simulink model "HEV_powersplit_adapted"  (R2026a)
settings: Solver=VariableStepAuto  StopTime=DriveCycles(Drive_Cycle_Num).time(end)  FixedStep=Ts  AbsTol=1e-3  EnableMultiTasking=on
PreLoadFcn:
  | mdlDir = fileparts(get_param(bdroot,'FileName'));
  | if exist(mdlDir,'dir'), addpath(genpath(mdlDir)); end;
  | HEV_Model_HomeDir = mdlDir;
  | decimation = 1;
  | HEV_Model_PARAM;
  | HEV_SeriesParallel_param_detailed;
StartFcn:
  | tic;
StopFcn:
  | Elapsed_Sim_Time = toc;
undefined symbols (not defined in the file): AH, AH0, Drive_Cycle_Num, HEV_Param, Ld, Lq, p, psim, System, Ts, Vbat, VDC_VECT
libraries: fl_lib x70, nesl_utility x54, ee_lib x10, sdl_lib x6, eeTransforms x4, eePmsmCurrentController x2, eeGeneralControl x2, eePmsmCurrentReferenceGen x2, eePwmGeneratorTwoLevel x2, batteryecm_lib x1, Capacitors_lib x1, eePmsmTorqueEstimator x1
(part 2 of 3)

== system HEV_powersplit_adapted/Power Split Device/Sensor Carrier Shaft ==
  Ideal Rotational Motion Sensor : fl_lib/Mechanical/Mechanical Sensors/Ideal Rotational Motion Sensor  reference=foundation.enum.MeasurementReference.difference  acceleration_port=false  velocity_port=true  position_port=true  wrap_angle=simscape.enum.onoff.off  offset=0 rad
  Ideal Torque Sensor : fl_lib/Mechanical/Mechanical Sensors/Ideal Torque Sensor
  Mechanical Rotational Reference : fl_lib/Mechanical/Rotational Elements/Mechanical Rotational Reference
  PS-Simulink Converter : nesl_utility/PS-Simulink Converter  PhysicalDomain=network_engine_domain  SubClassName=ps_output  LeftPortType=input  RightPortType=output  PseudoPeriodic=off  Frequencies=[]  VectorFormat=1-D array  Unit=N*m  AffineConversion=off
  PS-Simulink Converter1 : nesl_utility/PS-Simulink Converter  PhysicalDomain=network_engine_domain  SubClassName=ps_output  LeftPortType=input  RightPortType=output  PseudoPeriodic=off  Frequencies=[]  VectorFormat=1-D array  Unit=rad/s  AffineConversion=off
  PG : PMIOPort  Side=Right
  Sh : PMIOPort  Port=2  Side=Left
  tag scope: Carrier_Spd_radps=global, Carrier_Trq_Nm=global
  wires:
  PS-Simulink Converter/1 -> [Carrier_Trq_Nm]  "Carrier torque (Nm)"
  PS-Simulink Converter1/1 -> [Carrier_Spd_radps]
  connections:
  Ideal Torque Sensor/RConn1 -- Sh/RConn1 -- Ideal Rotational Motion Sensor/RConn1
  Mechanical Rotational Reference/LConn1 -- Ideal Rotational Motion Sensor/LConn1
  PS-Simulink Converter/LConn1 -- Ideal Torque Sensor/RConn2
  PS-Simulink Converter1/LConn1 -- Ideal Rotational Motion Sensor/RConn2
  PG/RConn1 -- Ideal Torque Sensor/LConn1

== system HEV_powersplit_adapted/Power Split Device/Sensor Ring Shaft ==
  Ideal Rotational Motion Sensor : fl_lib/Mechanical/Mechanical Sensors/Ideal Rotational Motion Sensor  reference=foundation.enum.MeasurementReference.difference  acceleration_port=false  velocity_port=true  position_port=true  wrap_angle=simscape.enum.onoff.off  offset=0 rad
  Ideal Torque Sensor : fl_lib/Mechanical/Mechanical Sensors/Ideal Torque Sensor
  Mechanical Rotational Reference : fl_lib/Mechanical/Rotational Elements/Mechanical Rotational Reference
  PS-Simulink Converter : nesl_utility/PS-Simulink Converter  PhysicalDomain=network_engine_domain  SubClassName=ps_output  LeftPortType=input  RightPortType=output  PseudoPeriodic=off  Frequencies=[]  VectorFormat=1-D array  Unit=N*m  AffineConversion=off
  PS-Simulink Converter1 : nesl_utility/PS-Simulink Converter  PhysicalDomain=network_engine_domain  SubClassName=ps_output  LeftPortType=input  RightPortType=output  PseudoPeriodic=off  Frequencies=[]  VectorFormat=1-D array  Unit=rad/s  AffineConversion=off
  PG : PMIOPort  Side=Right
  Sh : PMIOPort  Port=2  Side=Left
  tag scope: Ring_Spd_radps=global, Ring_Trq_Nm=global
  wires:
  PS-Simulink Converter/1 -> [Ring_Trq_Nm]  "Ring  torque (Nm)"
  PS-Simulink Converter1/1 -> [Ring_Spd_radps]  "Ring speed (rad/s)"
  connections:
  Ideal Rotational Motion Sensor/RConn1 -- PG/RConn1 -- Ideal Torque Sensor/RConn1
  Sh/RConn1 -- Ideal Torque Sensor/LConn1
  PS-Simulink Converter/LConn1 -- Ideal Torque Sensor/RConn2
  Mechanical Rotational Reference/LConn1 -- Ideal Rotational Motion Sensor/LConn1
  PS-Simulink Converter1/LConn1 -- Ideal Rotational Motion Sensor/RConn2

== system HEV_powersplit_adapted/Power Split Device/Sensor Sun Shaft ==
  Ideal Rotational Motion Sensor : fl_lib/Mechanical/Mechanical Sensors/Ideal Rotational Motion Sensor  reference=foundation.enum.MeasurementReference.difference  acceleration_port=false  velocity_port=true  position_port=true  wrap_angle=simscape.enum.onoff.off  offset=0 rad
  Ideal Torque Sensor : fl_lib/Mechanical/Mechanical Sensors/Ideal Torque Sensor
  Mechanical Rotational Reference : fl_lib/Mechanical/Rotational Elements/Mechanical Rotational Reference
  PS-Simulink Converter : nesl_utility/PS-Simulink Converter  PhysicalDomain=network_engine_domain  SubClassName=ps_output  LeftPortType=input  RightPortType=output  PseudoPeriodic=off  Frequencies=[]  VectorFormat=1-D array  Unit=N*m  AffineConversion=off
  PS-Simulink Converter1 : nesl_utility/PS-Simulink Converter  PhysicalDomain=network_engine_domain  SubClassName=ps_output  LeftPortType=input  RightPortType=output  PseudoPeriodic=off  Frequencies=[]  VectorFormat=1-D array  Unit=rad/s  AffineConversion=off
  PG : PMIOPort  Side=Right
  Sh : PMIOPort  Port=2  Side=Left
  tag scope: Sun_Spd_radps=global, Sun_Trq_Nm=global
  wires:
  PS-Simulink Converter1/1 -> [Sun_Spd_radps]
  PS-Simulink Converter/1 -> [Sun_Trq_Nm]  "Sun_Trq_Nm"
  connections:
  Sh/RConn1 -- Ideal Torque Sensor/LConn1
  PS-Simulink Converter1/LConn1 -- Ideal Rotational Motion Sensor/RConn2
  PS-Simulink Converter/LConn1 -- Ideal Torque Sensor/RConn2
  Mechanical Rotational Reference/LConn1 -- Ideal Rotational Motion Sensor/LConn1
  PG/RConn1 -- Ideal Torque Sensor/RConn1 -- Ideal Rotational Motion Sensor/RConn1

== system HEV_powersplit_adapted/Scopes/Drivetrain Scopes ==
  Speed (rad/s) : Scope  NumInputPorts=3
      settings: ActiveDisplayYMinimum=-100  ActiveDisplayYMaximum=500  DataLoggingMaxPoints=100  DataLoggingDecimation=decimation  DataLoggingVariableName=ScopeData2
  Torque (Nm) : Scope  Commented=on  NumInputPorts=3
      settings: ActiveDisplayYMinimum=-50  ActiveDisplayYMaximum=150  DataLoggingMaxPoints=100  DataLoggingDecimation=decimation  DataLoggingVariableName=ScopeData4
  wires:
  [Ring_Spd_radps] -> Speed (rad/s)/2  "Ring speed (rad/s) - motor"
  [Sun_Spd_radps] -> Speed (rad/s)/3  "Sun speed (rad/s) - generator"
  [Ring_Trq_Nm] -> Torque (Nm)/2  "Ring torque (Nm) - motor"
  [Carrier_Spd_radps] -> Speed (rad/s)/1  "Carrier speed (rad/s) - engine (ICE)"
  [Sun_Trq_Nm] -> Torque (Nm)/3  "Sun torque (Nm) - generator"
  [Carrier_Trq_Nm] -> Torque (Nm)/1  "Carrier torque (Nm) - engine (ICE)"

== system HEV_powersplit_adapted/Scopes/Power Calculation2 ==
  Spd : Inport
  Tq : Inport  Port=2
  Gain4 : Gain  Gain=1/1000
  Product2 : Product
  rpm2rad/s : Gain  Gain=pi/30
  Power : Outport  VectorParamsAs1DForOutWhenUnconnected=off
  wires:
  Spd/1 -> rpm2rad/s/1
  Gain4/1 -> Power/1
  Product2/1 -> Gain4/1
  Tq/1 -> Product2/2
  rpm2rad/s/1 -> Product2/1

== system HEV_powersplit_adapted/Scopes/Power Calculation ==
  Spd : Inport
  Tq : Inport  Port=2
  Gain4 : Gain  Gain=1/1000
  Product2 : Product
  rpm2rad/s : Gain  Gain=pi/30
  Power : Outport  VectorParamsAs1DForOutWhenUnconnected=off
  wires:
  Spd/1 -> rpm2rad/s/1
  Gain4/1 -> Power/1
  Product2/1 -> Gain4/1
  Tq/1 -> Product2/2
  rpm2rad/s/1 -> Product2/1

== system HEV_powersplit_adapted/Vehicle/Sensor Speed and Power ==
  Ideal Rotational Motion Sensor : fl_lib/Mechanical/Mechanical Sensors/Ideal Rotational Motion Sensor  reference=foundation.enum.MeasurementReference.difference  acceleration_port=false  velocity_port=true  position_port=true  wrap_angle=simscape.enum.onoff.off  offset=0 rad
  Ideal Torque Sensor : fl_lib/Mechanical/Mechanical Sensors/Ideal Torque Sensor
  Mechanical Rotational Reference : fl_lib/Mechanical/Rotational Elements/Mechanical Rotational Reference
  PS-Simulink Converter : nesl_utility/PS-Simulink Converter  PhysicalDomain=network_engine_domain  SubClassName=ps_output  LeftPortType=input  RightPortType=output  PseudoPeriodic=off  Frequencies=[]  VectorFormat=1-D array  Unit=N*m  AffineConversion=off
  PS-Simulink Converter1 : nesl_utility/PS-Simulink Converter  PhysicalDomain=network_engine_domain  SubClassName=ps_output  LeftPortType=input  RightPortType=output  PseudoPeriodic=off  Frequencies=[]  VectorFormat=1-D array  Unit=rad/s  AffineConversion=off
  Product : Product  RndMeth=Zero
  W2kW : Gain  Gain=0.001
  B : PMIOPort  Side=Left
  F : PMIOPort  Port=2  Side=Right
  tag scope: P_dem=global
  wires:
  W2kW/1 -> [P_dem]
  Product/1 -> W2kW/1
  PS-Simulink Converter/1 -> Product/1
  PS-Simulink Converter1/1 -> Product/2
  connections:
  Mechanical Rotational Reference/LConn1 -- Ideal Rotational Motion Sensor/RConn1
  Ideal Rotational Motion Sensor/LConn1 -- F/RConn1 -- Ideal Torque Sensor/RConn1
  B/RConn1 -- Ideal Torque Sensor/LConn1
  PS-Simulink Converter/LConn1 -- Ideal Torque Sensor/RConn2
  PS-Simulink Converter1/LConn1 -- Ideal Rotational Motion Sensor/RConn2

== system HEV_powersplit_adapted/Control/Engine Speed Controller/Engine Running ==
  note: Manual enable for control logic
  ICE_Enable : Inport
  Constant : Constant
  Select Logic : ManualSwitch  CurrentSetting=0
  Engine Running : Outport  VectorParamsAs1DForOutWhenUnconnected=off
  tag scope: engine_running=global
  wires:
  ICE_Enable/1 -> Select Logic/2
  Select Logic/1 -> Engine Running/1, [engine_running]
  Constant/1 -> Select Logic/1

== system HEV_powersplit_adapted/Control/Generator Controller/Enable Torque Demand ==
  Gen_Enable : Inport
  TrqDemCtrl : Inport  Port=2
  20Hz Lowpass Filter : TransferFcn  Denominator=[1/(2*pi*20) 1]
  Product : Product  RndMeth=Zero
  Select Logic : ManualSwitch  CurrentSetting=0
  G_Trq_Dem : Outport  VectorParamsAs1DForOutWhenUnconnected=off
  wires:
  Gen_Enable/1 -> 20Hz Lowpass Filter/1
  TrqDemCtrl/1 -> Product/2, Select Logic/2
  20Hz Lowpass Filter/1 -> Product/1
  Select Logic/1 -> G_Trq_Dem/1
  Product/1 -> Select Logic/1

== system HEV_powersplit_adapted/Control/Generator Controller/Speed controller ==
  note: This loop controls motor speed. The maximum value for V_wref is 5 volts,
      | which is equivalent to a speed demand of 10000rpm.
  Wref : Inport
  W : Inport  Port=2
  20Hz Lowpass Filter : TransferFcn  Denominator=[1/(2*pi*20) 1]
  Gen RPM to V : Gain  Gain=5/10000
  Ki : Gain  Gain=HEV_Param.Control.Gen.Ki
  Kp : Gain  Gain=HEV_Param.Control.Gen.Kp
  Limits [-5,5] : Integrator  ExternalReset=either  LimitOutput=on  UpperSaturationLimit=5  LowerSaturationLimit=-5
  Sum : Sum  Inputs=-+|
  Sum1 : Sum  Inputs=++|
  Volts/Nm : Gain  Gain=400/5
  "[-5,5]" : Saturate  UpperLimit=5  LowerLimit=-5
  rpm2volts : Gain  Gain=5/10000
  Tref : Outport  VectorParamsAs1DForOutWhenUnconnected=off
  wires:
  Sum/1 -> Ki/1, Kp/1
  [engine_running] -> Limits [-5,5]/2
  20Hz Lowpass Filter/1 -> Sum/1
  Limits [-5,5]/1 -> Sum1/1
  Kp/1 -> Sum1/2
  Ki/1 -> Limits [-5,5]/1
  Sum1/1 -> "[-5,5]"/1
  W/1 -> Gen RPM to V/1
  Wref/1 -> rpm2volts/1
  "[-5,5]"/1 -> Volts/Nm/1
  rpm2volts/1 -> Sum/2
  Gen RPM to V/1 -> 20Hz Lowpass Filter/1
  Volts/Nm/1 -> Tref/1

== system HEV_powersplit_adapted/Control/Generator Controller/Subsystem1 ==
  In1 : Inport
  Gen_RPM_Dem : Outport  VectorParamsAs1DForOutWhenUnconnected=off
  wires:
  In1/1 -> Gen_RPM_Dem/1

== system HEV_powersplit_adapted/Control/Motor Controller/Enable Torque Demand ==
  Mot_Enable : Inport
  TrqDemCtrl : Inport  Port=2
  20Hz Lowpass Filter : TransferFcn  Commented=on  Denominator=[1/(2*pi*10) 1]
  Product : Product  RndMeth=Zero
  Select Logic : ManualSwitch  CurrentSetting=0
  TrqDem : Outport  VectorParamsAs1DForOutWhenUnconnected=off
  wires:
  Mot_Enable/1 -> 20Hz Lowpass Filter/1
  TrqDemCtrl/1 -> Product/2, Select Logic/2
  Product/1 -> Select Logic/1
  20Hz Lowpass Filter/1 -> Product/1
  Select Logic/1 -> TrqDem/1

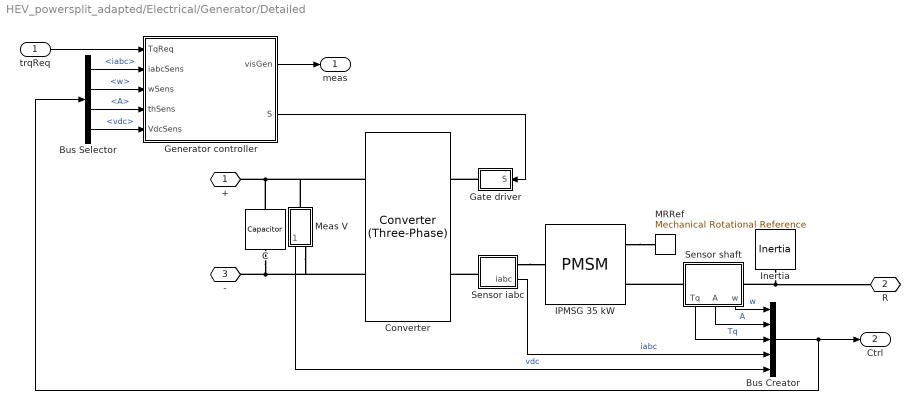
== system HEV_powersplit_adapted/Electrical/Generator/Detailed ==
  trqReq : Inport
  Bus Creator : BusCreator  Inputs=5
  Bus Selector : BusSelector  OutputSignals=iabc,w,A,vdc
  C : fl_lib/Electrical/Electrical Elements/Capacitor  c=Cdc F  r=1e-6 Ohm  g=0 1/Ohm  i_specify=off  i_priority=None  i=0 A  i_nominal_specify=off  i_nominal_value=1  i_nominal_unit=A  v_specify=off  v_priority=None  v=0 V  v_nominal_specify=off  v_nominal_value=1  v_nominal_unit=V  vc_specify=on  vc_priority=None  vc=Vbat*1.4 V  vc_nominal_specify=off  vc_nominal_value=1  vc_nominal_unit=V
  Converter : ee_lib/Semiconductors & Converters/Converters/Converter (Three-Phase)  port_option=ee.enum.threePhasePort.composite  fidelity_option=ee.enum.converters.fidelity.detailed  device_type=2  showThermalPort=false  K=0  Vth=0.5 V  Vgt=1 V  Vgt_off=-1 V  Ih=1 A  Vf=0.8 V  Ron=0.001 Ohm  Rds=0.001 Ohm  Goff=1e-5 1/Ohm  Eon_scalar=22.86e-3 J  Eoff_scalar=17.14e-3 J  Eoff_natural_commutation=10e-3 J  Voff=300 V  Iout_scalar=600 A  onCurrentMeasDelay=0 s  useCurrentFromPreviousCycle=false  useVoltageFromPreviousCycle=false  diode_param=2  diode_Vf=0.8 V  diode_Ron=0.001 Ohm  diode_Goff=1e-5 1/Ohm  diode_C=50 nF  diode_iRM=-235 A  diode_iF=300 A  diode_idot=-50 A/us  diode_trr_param=1  diode_trr_factor=3  diode_trr=15 us  diode_Qrr=1.5e+3 s*uA  diode_rec_loss_model=ee.enum.diode.reverseRecoveryModel.fixed  diode_ErecVal=0 J  diode_scaleWithIandV=false  diode_ErecMat=zeros(2, 3) J  diode_TjrecVec=[298.15, 398.15] K  diode_IfrecVec=[.1, 1, 10] A  diode_IrecVal=10 A  diode_VrecVal=10 V  diode_tFilter=1 / 1000 / 100 s  thermal_network_parameterization=ee.enum.thermalNetworkTopology.external  Rth=[.08, .5] K/W  Rth_Cauer=[.08, .1, .5] K/W  Rth_Foster=[.08, .14, .22, .16] K/W  thermal_mass_parameterization=ee.enum.thermalNetwork.timeconstant  thermal_mass=[.01, .5] J/K  thermal_mass_Cauer=[.01, .1, .5] J/K  thermal_mass_Foster=[.001, .005, .05, .5] J/K  thermal_time_constant=[.001, .2] s  thermal_time_constant_Cauer=[.001, .1, .2] s  thermal_time_constant_Foster=[7e-05, .0007, .01, .08] s  thermal_mass_initial_temperatures=[25, 25] degC  thermal_mass_initial_temperatures_Cauer=[25, 25, 25] degC  junction_thermal_mass=0.01 J/K  Tvec_initial_Foster=[25, 25, 25, 25] degC  snubber_type=0  Cs=1e-7 F  Rs=0.1 Ohm  Vce_loss=[0, 150, 300] V
      settings: LogSimulationData=on
  Gate driver : Subsystem
  Generator controller : Subsystem
  IPMSG 35 kW : ee_lib/Electromechanical/Permanent Magnet/PMSM  port_option=ee.enum.threePhasePort.composite  winding_type=ee.enum.statorconnection.wye  machine_param=ee.enum.pmsm.parameterization.constant  nPolePairs=p  pmflux_param=1  pm_flux_linkage=psim Wb  torque_constant=0.18 N*m/A  back_emf_constant=0.18 V/(rad/s)  stator_param=1  Ld=Ld H  Lq=Lq H  idVec=[-200, 0, 200] A  iqVec=[-200, 0, 200] A  LdMatrix=0.0002 * ones(3, 3) H  LqMatrix=0.0002 * ones(3, 3) H  PmMatrix=0.1 * ones(3, 3) Wb  ktMatrix=0.18 * ones(3, 3) N*m/A  keMatrix=0.18 * ones(3, 3) V/(rad/s)  L0=L0 H  Ls=0.0002 H  Lm=0.00002 H  Ms=0.00002 H  Rs=Rs Ohm  zero_sequence=ee.enum.park.zerosequence.exclude  axes_param=1  loss_param=ee.enum.ironloss.none  losses_oc=[0, 0, 0] W  losses_sc=[0, 0, 0] W  f_losses=60 Hz  Isc_losses=95 A  J=0.01 kg*m^2  lam=0 N*m/(rad/s)  i_d_specify=off  i_d_priority=None  i_d=0 A  i_d_nominal_specify=off  i_d_nominal_value=1  i_d_nominal_unit=A  i_q_specify=off  i_q_priority=None  i_q=0 A  i_q_nominal_specify=off  i_q_nominal_value=1  i_q_nominal_unit=A  torque_specify=off  torque_priority=None  torque=0 N*m  torque_nominal_specify=off  torque_nominal_value=1  torque_nominal_unit=N*m  angular_velocity_specify=on  angular_velocity_priority=Low  angular_velocity=0 rpm  angular_velocity_nominal_specify=off  angular_velocity_nominal_value=1  angular_velocity_nominal_unit=rpm  angular_position_specify=off  angular_position_priority=None  angular_position=0 deg  angular_position_nominal_specify=off  angular_position_nominal_value=1  angular_position_nominal_unit=deg  alpha=3.93e-3 1/K  alpha_flux=-0.001 1/K  Tmeas=298.15 K  stator_thermal_mass=100 J/K  rotor_thermal_mass=200 J/K  Rm_percent_rotor=90  Rd_percent_rotor=30  temperatureA_specify=off  temperatureA_priority=High  temperatureA=25 degC  temperatureA_nominal_specify=off  temperatureA_nominal_value=1  temperatureA_nominal_unit=degC  temperatureB_specify=off  temperatureB_priority=High  temperatureB=25 degC  temperatureB_nominal_specify=off  temperatureB_nominal_value=1  temperatureB_nominal_unit=degC  temperatureC_specify=off  temperatureC_priority=High  temperatureC=25 degC  temperatureC_nominal_specify=off  temperatureC_nominal_value=1  temperatureC_nominal_unit=degC  temperatureR_specify=off  temperatureR_priority=High  temperatureR=25 degC  temperatureR_nominal_specify=off  temperatureR_nominal_value=1  temperatureR_nominal_unit=degC
      settings: LogSimulationData=on  InternalSimscapePortConfiguration="{\"Bottom\":[],\"Left\":[{\"id\":\"N\",\"label\":\"~\",\"type\":\"foundation.electrical.three_phase\"}],\"Right\":[{\"id\":\"R\",\"label\":\"R\",\"type\":\"foundation.mechanical.rotational.rotational\"},{\"id\":\"C\",\"label\":\"C\",\"type\":\"foundation.mechanical.rotational.rotational\"}],\"Top\":[]}"
  Inertia : fl_lib/Mechanical/Rotational Elements/Inertia  inertia=0.1 kg*m^2  num_ports=foundation.enum.numPorts2.one  w_specify=on  w_priority=Low  w=0 rad/s  w_nominal_specify=off  w_nominal_value=1  w_nominal_unit=rad/s  t_specify=off  t_priority=None  t=0 N*m  t_nominal_specify=off  t_nominal_value=1  t_nominal_unit=N*m
  MRRef : fl_lib/Mechanical/Rotational Elements/Mechanical Rotational Reference
  Meas V : Subsystem
  Sensor iabc : Subsystem
      settings: PortSchema="{\"entries\":[{\"content\":{\"sides\":[{\"content\":{\"connectorIds\":[\"LConn1\"]},\"type\":\"ConnectorPlacement.EquallySpacedRectSide\",\"uuid\":\"bc3757cc-4537-444e-89af-7b7d8c8c1fa7\"},{\"content\":{\"connectorIds\":[\"RConn1\",\"Out1\"],\"side\":\"RIGHT\"},\"type\":\"ConnectorPlacement.EquallySpacedRectSide\",\"uuid\":\"908bf4c4-26f6-4d8a-bcf8-68236027f5f8\"},{\"content\":{\"connectorIds\":[],\"side\":\"TOP\"},\"type\":\"ConnectorPlacement.EquallySpacedRectSide\",\"uuid\":\"33f228db-ba47-4718-96dc-a72de309ae8c\"}]},\"type\":\"ConnectorPlacement.EquallySpacedConnector\",\"uuid\":\"345f3578-0572-4e64-b2f3-84728129a12d\"}],\"packageUris\":[\"http://schema.mathworks.com/mf0/Connector/R2020b\"],\"version\":\"1.0\"}"
  Sensor shaft : Subsystem
      settings: PortSchema="{\"entries\":[{\"content\":{\"sides\":[{\"content\":{\"connectorIds\":[\"LConn1\"]},\"type\":\"ConnectorPlacement.EquallySpacedRectSide\",\"uuid\":\"0db9bac0-0ae1-4d98-a677-466f391c258c\"},{\"content\":{\"connectorIds\":[\"RConn1\"],\"side\":\"RIGHT\"},\"type\":\"ConnectorPlacement.EquallySpacedRectSide\",\"uuid\":\"8934243c-3b81-4e7c-b06c-d9d72f311b85\"},{\"content\":{\"connectorIds\":[],\"side\":\"TOP\"},\"type\":\"ConnectorPlacement.EquallySpacedRectSide\",\"uuid\":\"85d02103-2e2c-4b6a-97e8-ffc8c956f28d\"},{\"content\":{\"connectorIds\":[\"Out1\",\"Out2\",\"Out3\"],\"side\":\"BOTTOM\"},\"type\":\"ConnectorPlacement.EquallySpacedRectSide\",\"uuid\":\"2e7d2385-134f-4bd8-b3f4-60582ce11538\"}]},\"type\":\"ConnectorPlacement.EquallySpacedConnector\",\"uuid\":\"45a37dc1-16bf-4b9c-909e-727af625c5bc\"}],\"packageUris\":[\"http://schema.mathworks.com/mf0/Connector/R2020b\"],\"version\":\"1.0\"}"
  + : PMIOPort  Side=Left
  R : PMIOPort  Port=2  Side=Right
  - : PMIOPort  Port=3  Side=Left
  meas : Outport
  Ctrl : Outport  Port=2
  wires:
  Generator controller/1(visGen) -> meas/1
  trqReq/1 -> Generator controller/1(TqReq)
  Bus Selector/2 -> Generator controller/3(wSens)  "<w>"
  Bus Selector/4 -> Generator controller/5(VdcSens)  "<vdc>"
  Bus Selector/3 -> Generator controller/4(thSens)  "<A>"
  Bus Selector/1 -> Generator controller/2(iabcSens)  "<iabc>"
  Bus Creator/1 -> Bus Selector/1, Ctrl/1
  Sensor shaft/1(Tq) -> Bus Creator/3  "Tq"
  Sensor iabc/1(iabc) -> Bus Creator/4  "iabc"
  Meas V/1(Vdc) -> Bus Creator/5  "vdc"
  Sensor shaft/3(w) -> Bus Creator/1  "w"
  Sensor shaft/2(A) -> Bus Creator/2  "A"
  Generator controller/2(S) -> Gate driver/1(S)
  connections:
  C/LConn1 -- Meas V/LConn1 -- Converter/RConn1 -- +/RConn1
  Sensor iabc/RConn1 -- IPMSG 35 kW/LConn1
  Sensor iabc/LConn1 -- Converter/LConn2
  Inertia/LConn1 -- R/RConn1 -- Sensor shaft/RConn1
  Sensor shaft/LConn1 -- IPMSG 35 kW/RConn1
  Gate driver/RConn1 -- Converter/LConn1
  C/RConn1 -- -/RConn1 -- Converter/RConn2 -- Meas V/RConn1
  IPMSG 35 kW/RConn2 -- MRRef/LConn1

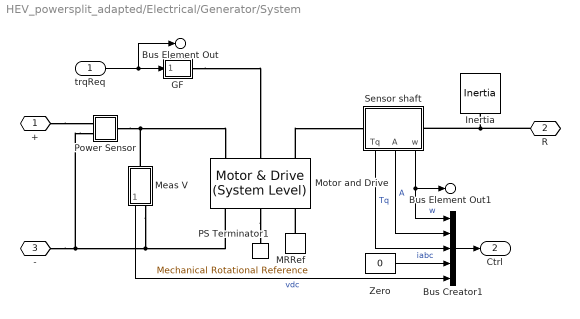
== system HEV_powersplit_adapted/Electrical/Generator/System ==
  trqReq : Inport
  Bus Creator1 : BusCreator  Inputs=5
  GF : Subsystem
      mask Display: disp('GF')
  Inertia : fl_lib/Mechanical/Rotational Elements/Inertia  inertia=HEV_Param.Generator.Shaft_Inertia kg*m^2  num_ports=foundation.enum.numPorts2.one  w_specify=on  w_priority=None  w=0 rad/s  w_nominal_specify=off  w_nominal_value=1  w_nominal_unit=rad/s  t_specify=off  t_priority=High  t=0 N*m  t_nominal_specify=off  t_nominal_value=1  t_nominal_unit=N*m
  MRRef : fl_lib/Mechanical/Rotational Elements/Mechanical Rotational Reference
  Meas V : Subsystem
  Motor and Drive : ee_lib/Electromechanical/Motor & Drive (System Level)  torque_speed_param=1  overtorque_param=ee.enum.electromech.overtorque.no  T_t=HEV_Param.Generator.TorqSpdLUT.TorqueNm N*m  T_t_intermittent=[.36, .32, .28, 0] N*m  T_t_2D=[.09, .09, .09; .08, .08, .08; .07, .07, .07; 0, 0, 0] N*m  T_t_intermittent_2D=[.36, .36, .36; .32, .32, .32; .28, .28, .28; 0, 0, 0] N*m  w_t=HEV_Param.Generator.TorqSpdLUT.SpeedRPM rpm  vdc_t=[6, 12, 24] V  torque_max=0.1 N*m  power_max=30 W  torque_max_intermittent=0.4 N*m  power_max_intermittent=120 W  time_overtorque=30 s  time_recover=60 s  Tc=HEV_Param.Generator.TorqueControl_TimeConst/2 s  EnableSwitch=simscape.enum.onoff.off  losses_param=1  eff=90  w_eff=2000 rpm  T_eff=200 N*m  Piron=0 W  Pbase=HEV_Param.Generator.TorqIndep_Elec_Loss W  w_eff_vec=[-8000 -4000 0 4000 8000] rpm  T_eff_vec=[0 0.03 0.06 0.09] N*m  v_eff_vec=[100, 250, 400] V  losses_mat=[1.49 1.67 2.21 3.10; 0.42 0.69 1.14 2.03; 0.06 0.24 0.78 1.68; 0.42 0.69 1.14 2.03; 1.49 1.67 2.21 3.10] W  efficiency_mat=[95 95 95 95; 95 95 95 95; 95 95 95 95; 95 95 95 95; 95 95 95 95]  losses_mat_3D=ones(5, 4, 3) W  efficiency_mat_3D=95 * ones(5, 4, 3)  Res=HEV_Param.Generator.Series_Resistance Ohm  J=0 kg*m^2  lam=HEV_Param.Generator.Damping N*m/(rad/s)  speed0=0 rpm  faulted_specify=off  faulted_priority=None  faulted=0  faulted_nominal_specify=off  faulted_nominal_value=1  faulted_nominal_unit=1  isSwitchedOff_specify=off  isSwitchedOff_priority=None  isSwitchedOff=0  isSwitchedOff_nominal_specify=off  isSwitchedOff_nominal_value=1  isSwitchedOff_nominal_unit=1  torqueLimitContinuous_specify=off  torqueLimitContinuous_priority=None  torqueLimitContinuous=0 N*m  torqueLimitContinuous_nominal_specify=off  torqueLimitContinuous_nominal_value=1  torqueLimitContinuous_nominal_unit=N*m  TabulateLossesForMultipleTemperatures=false  alpha=3.93e-3 1/K  Tmeas=25 degC  TmeasVec=[25, 75, 125] degC  Tmeas2=125 degC  losses_mat_T2=[1.49, 1.74, 2.49, 3.74; .42, .67, 1.42, 2.67; .06, .31, 1.06, 2.31; .42, .67, 1.42, 2.67; 1.49, 1.74, 2.49, 3.74] W  efficiency_mat_T2=[95, 95, 95, 95; 95, 95, 95, 95; 95, 95, 95, 95; 95, 95, 95, 95; 95, 95, 95, 95]  losses_mat_3D_T2=ones(5, 4, 3) W  efficiency_mat_3D_T2=95 * ones(5, 4, 3)  lossesMatMultipleTemperatures=ones(5, 4, 3) W  efficiencyMatMultipleTemperatures=95 * ones(5, 4, 3)  lossesMat4DMultipleTemperatures=ones(5, 4, 3, 3) W  efficiencyMat4DMultipleTemperatures=95 * ones(5, 4, 3, 3)  thermal_mass=100 J/K  initial_temperature=25 degC
  PS Terminator1 : fl_lib/Physical Signals/Sinks/PS Terminator
  Power Sensor : Subsystem
      mask Display: disp('S')
  Sensor shaft : Subsystem
      settings: PortSchema="{\"entries\":[{\"content\":{\"sides\":[{\"content\":{\"connectorIds\":[\"LConn1\"]},\"type\":\"ConnectorPlacement.EquallySpacedRectSide\",\"uuid\":\"0db9bac0-0ae1-4d98-a677-466f391c258c\"},{\"content\":{\"connectorIds\":[\"RConn1\"],\"side\":\"RIGHT\"},\"type\":\"ConnectorPlacement.EquallySpacedRectSide\",\"uuid\":\"8934243c-3b81-4e7c-b06c-d9d72f311b85\"},{\"content\":{\"side\":\"TOP\"},\"type\":\"ConnectorPlacement.EquallySpacedRectSide\",\"uuid\":\"85d02103-2e2c-4b6a-97e8-ffc8c956f28d\"},{\"content\":{\"connectorIds\":[\"Out1\",\"Out2\",\"Out3\"],\"side\":\"BOTTOM\"},\"type\":\"ConnectorPlacement.EquallySpacedRectSide\",\"uuid\":\"2e7d2385-134f-4bd8-b3f4-60582ce11538\"}]},\"type\":\"ConnectorPlacement.EquallySpacedConnector\",\"uuid\":\"45a37dc1-16bf-4b9c-909e-727af625c5bc\"}],\"packageUris\":[\"http://schema.mathworks.com/mf0/Connector/R2020b\"],\"version\":\"1.0\"}"
  Zero : Constant  Value=0  OutDataTypeStr=Inherit: Inherit via back propagation
  + : PMIOPort  Side=Left
  R : PMIOPort  Port=2  Side=Right
  - : PMIOPort  Port=3  Side=Left
  Bus Element Out : Outport  PortName=meas  Element=TqRef
  Bus Element Out1 : Outport  PortName=meas  Element=Spd
  Ctrl : Outport  Port=2  VectorParamsAs1DForOutWhenUnconnected=off
  wires:
  Meas V/1(Vdc) -> Bus Creator1/5  "vdc"
  Bus Creator1/1 -> Ctrl/1
  Sensor shaft/3(w) -> Bus Element Out1/1, Bus Creator1/1  "w"
  Zero/1 -> Bus Creator1/4  "iabc"
  Sensor shaft/1(Tq) -> Bus Creator1/3  "Tq"
  Sensor shaft/2(A) -> Bus Creator1/2  "A"
  trqReq/1 -> Bus Element Out/1, GF/1(In1)
  connections:
  R/RConn1 -- Sensor shaft/RConn1 -- Inertia/LConn1
  Power Sensor/LConn2 -- -/RConn1 -- Motor and Drive/RConn1 -- Meas V/RConn1
  +/RConn1 -- Power Sensor/LConn1
  Power Sensor/RConn1 -- Motor and Drive/LConn1 -- Meas V/LConn1
  GF/RConn1 -- Motor and Drive/LConn2
  Motor and Drive/RConn2 -- PS Terminator1/LConn1
  MRRef/LConn1 -- Motor and Drive/RConn3
  Motor and Drive/LConn3 -- Sensor shaft/LConn1

== system HEV_powersplit_adapted/Electrical/Generic/Measurements1 ==
  Bus Creator : BusCreator  Inputs=4
  Calc Pct : Gain  Gain=1/AH*100
  Calculate battery power & charge : Subsystem
  Gain : Gain  Gain=1/100
  PS-Simulink Converter1 : nesl_utility/PS-Simulink Converter  PhysicalDomain=network_engine_domain  SubClassName=ps_output  LeftPortType=input  RightPortType=output  PseudoPeriodic=off  Frequencies=[]  VectorFormat=1-D array  Unit=V  AffineConversion=off
  PS-Simulink Converter2 : nesl_utility/PS-Simulink Converter  PhysicalDomain=network_engine_domain  SubClassName=ps_output  LeftPortType=input  RightPortType=output  PseudoPeriodic=off  Frequencies=[]  VectorFormat=1-D array  Unit=A  AffineConversion=off
  VBatt : PMIOPort  Side=Left
  IBatt : PMIOPort  Port=2  Side=Left
  Batt_Ah : Outport  VectorParamsAs1DForOutWhenUnconnected=off
  Batt_Meas : Outport  Port=2  VectorParamsAs1DForOutWhenUnconnected=off
  SOC : Outport  Port=3
  wires:
  Bus Creator/1 -> Batt_Meas/1
  PS-Simulink Converter2/1 -> Bus Creator/4  "Current (A)"
  PS-Simulink Converter1/1 -> Bus Creator/3  "Voltage (V)"
  Calc Pct/1 -> Gain/1, Bus Creator/2  "SOC (%)"
  Calculate battery power & charge/1(Ah) -> Batt_Ah/1, Calc Pct/1, Bus Creator/1  "Batt_Ah"
  Gain/1 -> SOC/1
  connections:
  PS-Simulink Converter2/LConn1 -- IBatt/RConn1 -- Calculate battery power & charge/LConn2
  PS-Simulink Converter1/LConn1 -- VBatt/RConn1 -- Calculate battery power & charge/LConn1

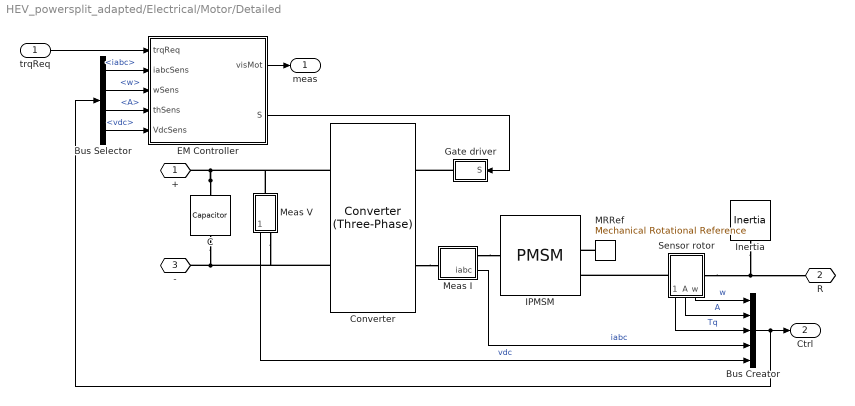
== system HEV_powersplit_adapted/Electrical/Motor/Detailed ==
  trqReq : Inport
  Bus Creator : BusCreator  Inputs=5
  Bus Selector : BusSelector  OutputSignals=iabc,w,A,vdc
  C : fl_lib/Electrical/Electrical Elements/Capacitor  c=Cdc F  r=1e-6 Ohm  g=0 1/Ohm  i_specify=off  i_priority=None  i=0 A  i_nominal_specify=off  i_nominal_value=1  i_nominal_unit=A  v_specify=off  v_priority=None  v=0 V  v_nominal_specify=off  v_nominal_value=1  v_nominal_unit=V  vc_specify=on  vc_priority=None  vc=Vbat*1.4 V  vc_nominal_specify=off  vc_nominal_value=1  vc_nominal_unit=V
  Converter : ee_lib/Semiconductors & Converters/Converters/Converter (Three-Phase)  port_option=ee.enum.threePhasePort.composite  fidelity_option=ee.enum.converters.fidelity.detailed  device_type=2  showThermalPort=false  K=0  Vth=0.5 V  Vgt=1 V  Vgt_off=-1 V  Ih=1 A  Vf=0.8 V  Ron=0.001 Ohm  Rds=0.001 Ohm  Goff=1e-5 1/Ohm  Eon_scalar=22.86e-3 J  Eoff_scalar=17.14e-3 J  Eoff_natural_commutation=10e-3 J  Voff=300 V  Iout_scalar=600 A  onCurrentMeasDelay=0 s  useCurrentFromPreviousCycle=false  useVoltageFromPreviousCycle=false  diode_param=2  diode_Vf=0.8 V  diode_Ron=0.001 Ohm  diode_Goff=1e-5 1/Ohm  diode_C=50 nF  diode_iRM=-235 A  diode_iF=300 A  diode_idot=-50 A/us  diode_trr_param=1  diode_trr_factor=3  diode_trr=15 us  diode_Qrr=1.5e+3 s*uA  diode_rec_loss_model=ee.enum.diode.reverseRecoveryModel.fixed  diode_ErecVal=0 J  diode_scaleWithIandV=false  diode_ErecMat=zeros(2, 3) J  diode_TjrecVec=[298.15, 398.15] K  diode_IfrecVec=[.1, 1, 10] A  diode_IrecVal=10 A  diode_VrecVal=10 V  diode_tFilter=1 / 1000 / 100 s  thermal_network_parameterization=ee.enum.thermalNetworkTopology.external  Rth=[.08, .5] K/W  Rth_Cauer=[.08, .1, .5] K/W  Rth_Foster=[.08, .14, .22, .16] K/W  thermal_mass_parameterization=ee.enum.thermalNetwork.timeconstant  thermal_mass=[.01, .5] J/K  thermal_mass_Cauer=[.01, .1, .5] J/K  thermal_mass_Foster=[.001, .005, .05, .5] J/K  thermal_time_constant=[.001, .2] s  thermal_time_constant_Cauer=[.001, .1, .2] s  thermal_time_constant_Foster=[7e-05, .0007, .01, .08] s  thermal_mass_initial_temperatures=[25, 25] degC  thermal_mass_initial_temperatures_Cauer=[25, 25, 25] degC  junction_thermal_mass=0.01 J/K  Tvec_initial_Foster=[25, 25, 25, 25] degC  snubber_type=0  Cs=1e-7 F  Rs=0.1 Ohm  Vce_loss=[0, 150, 300] V
      settings: LogSimulationData=on
  EM Controller : Subsystem
  Gate driver : Subsystem
  IPMSM : ee_lib/Electromechanical/Permanent Magnet/PMSM  port_option=ee.enum.threePhasePort.composite  winding_type=ee.enum.statorconnection.wye  machine_param=ee.enum.pmsm.parameterization.constant  nPolePairs=p  pmflux_param=1  pm_flux_linkage=psim Wb  torque_constant=0.18 N*m/A  back_emf_constant=0.18 V/(rad/s)  stator_param=1  Ld=Ld H  Lq=Lq H  idVec=[-200, 0, 200] A  iqVec=[-200, 0, 200] A  LdMatrix=0.0002 * ones(3, 3) H  LqMatrix=0.0002 * ones(3, 3) H  PmMatrix=0.1 * ones(3, 3) Wb  ktMatrix=0.18 * ones(3, 3) N*m/A  keMatrix=0.18 * ones(3, 3) V/(rad/s)  L0=L0 H  Ls=0.0002 H  Lm=0.00002 H  Ms=0.00002 H  Rs=Rs Ohm  zero_sequence=ee.enum.park.zerosequence.exclude  axes_param=1  loss_param=ee.enum.ironloss.none  losses_oc=[0, 0, 0] W  losses_sc=[0, 0, 0] W  f_losses=60 Hz  Isc_losses=95 A  J=0.01 kg*m^2  lam=0 N*m/(rad/s)  i_d_specify=off  i_d_priority=None  i_d=0 A  i_d_nominal_specify=off  i_d_nominal_value=1  i_d_nominal_unit=A  i_q_specify=off  i_q_priority=None  i_q=0 A  i_q_nominal_specify=off  i_q_nominal_value=1  i_q_nominal_unit=A  torque_specify=off  torque_priority=None  torque=0 N*m  torque_nominal_specify=off  torque_nominal_value=1  torque_nominal_unit=N*m  angular_velocity_specify=on  angular_velocity_priority=Low  angular_velocity=0 rpm  angular_velocity_nominal_specify=off  angular_velocity_nominal_value=1  angular_velocity_nominal_unit=rpm  angular_position_specify=off  angular_position_priority=None  angular_position=0 deg  angular_position_nominal_specify=off  angular_position_nominal_value=1  angular_position_nominal_unit=deg  alpha=3.93e-3 1/K  alpha_flux=-0.001 1/K  Tmeas=298.15 K  stator_thermal_mass=100 J/K  rotor_thermal_mass=200 J/K  Rm_percent_rotor=90  Rd_percent_rotor=30  temperatureA_specify=off  temperatureA_priority=High  temperatureA=25 degC  temperatureA_nominal_specify=off  temperatureA_nominal_value=1  temperatureA_nominal_unit=degC  temperatureB_specify=off  temperatureB_priority=High  temperatureB=25 degC  temperatureB_nominal_specify=off  temperatureB_nominal_value=1  temperatureB_nominal_unit=degC  temperatureC_specify=off  temperatureC_priority=High  temperatureC=25 degC  temperatureC_nominal_specify=off  temperatureC_nominal_value=1  temperatureC_nominal_unit=degC  temperatureR_specify=off  temperatureR_priority=High  temperatureR=25 degC  temperatureR_nominal_specify=off  temperatureR_nominal_value=1  temperatureR_nominal_unit=degC
      settings: AttributesFormatString=35 kW  LogSimulationData=on  InternalSimscapePortConfiguration="{\"Bottom\":[],\"Left\":[{\"id\":\"N\",\"label\":\"~\",\"type\":\"foundation.electrical.three_phase\"}],\"Right\":[{\"id\":\"R\",\"label\":\"R\",\"type\":\"foundation.mechanical.rotational.rotational\"},{\"id\":\"C\",\"label\":\"C\",\"type\":\"foundation.mechanical.rotational.rotational\"}],\"Top\":[]}"
  Inertia : fl_lib/Mechanical/Rotational Elements/Inertia  inertia=0.1 kg*m^2  num_ports=foundation.enum.numPorts2.one  w_specify=on  w_priority=Low  w=0 rad/s  w_nominal_specify=off  w_nominal_value=1  w_nominal_unit=rad/s  t_specify=off  t_priority=None  t=0 N*m  t_nominal_specify=off  t_nominal_value=1  t_nominal_unit=N*m
  MRRef : fl_lib/Mechanical/Rotational Elements/Mechanical Rotational Reference
  Meas I : Subsystem
      settings: PortSchema="{\"entries\":[{\"content\":{\"sides\":[{\"content\":{\"connectorIds\":[\"LConn1\"]},\"type\":\"ConnectorPlacement.EquallySpacedRectSide\",\"uuid\":\"bc3757cc-4537-444e-89af-7b7d8c8c1fa7\"},{\"content\":{\"connectorIds\":[\"RConn1\",\"Out1\"],\"side\":\"RIGHT\"},\"type\":\"ConnectorPlacement.EquallySpacedRectSide\",\"uuid\":\"908bf4c4-26f6-4d8a-bcf8-68236027f5f8\"},{\"content\":{\"connectorIds\":[],\"side\":\"TOP\"},\"type\":\"ConnectorPlacement.EquallySpacedRectSide\",\"uuid\":\"33f228db-ba47-4718-96dc-a72de309ae8c\"}]},\"type\":\"ConnectorPlacement.EquallySpacedConnector\",\"uuid\":\"345f3578-0572-4e64-b2f3-84728129a12d\"}],\"packageUris\":[\"http://schema.mathworks.com/mf0/Connector/R2020b\"],\"version\":\"1.0\"}"
  Meas V : Subsystem
  Sensor rotor : Subsystem
      settings: PortSchema="{\"entries\":[{\"content\":{\"sides\":[{\"content\":{\"connectorIds\":[\"LConn1\"]},\"type\":\"ConnectorPlacement.EquallySpacedRectSide\",\"uuid\":\"0db9bac0-0ae1-4d98-a677-466f391c258c\"},{\"content\":{\"connectorIds\":[\"RConn1\"],\"side\":\"RIGHT\"},\"type\":\"ConnectorPlacement.EquallySpacedRectSide\",\"uuid\":\"8934243c-3b81-4e7c-b06c-d9d72f311b85\"},{\"content\":{\"connectorIds\":[],\"side\":\"TOP\"},\"type\":\"ConnectorPlacement.EquallySpacedRectSide\",\"uuid\":\"85d02103-2e2c-4b6a-97e8-ffc8c956f28d\"},{\"content\":{\"connectorIds\":[\"Out1\",\"Out2\",\"Out3\"],\"side\":\"BOTTOM\"},\"type\":\"ConnectorPlacement.EquallySpacedRectSide\",\"uuid\":\"a4912837-dd6e-4716-a3b5-e9be70514ed9\"}]},\"type\":\"ConnectorPlacement.EquallySpacedConnector\",\"uuid\":\"45a37dc1-16bf-4b9c-909e-727af625c5bc\"}],\"packageUris\":[\"http://schema.mathworks.com/mf0/Connector/R2020b\"],\"version\":\"1.0\"}"
  + : PMIOPort  Side=Left
  R : PMIOPort  Port=2  Side=Right
  - : PMIOPort  Port=3  Side=Left
  meas : Outport
  Ctrl : Outport  Port=2
  wires:
  EM Controller/1(visMot) -> meas/1
  Bus Selector/3 -> EM Controller/4(thSens)  "<A>"
  Bus Selector/4 -> EM Controller/5(VdcSens)  "<vdc>"
  Bus Selector/1 -> EM Controller/2(iabcSens)  "<iabc>"
  Bus Creator/1 -> Ctrl/1, Bus Selector/1
  Bus Selector/2 -> EM Controller/3(wSens)  "<w>"
  trqReq/1 -> EM Controller/1(trqReq)
  Sensor rotor/1(Tq) -> Bus Creator/3  "Tq"
  Meas I/1(iabc) -> Bus Creator/4  "iabc"
  Meas V/1(Vdc) -> Bus Creator/5  "vdc"
  Sensor rotor/2(A) -> Bus Creator/2  "A"
  EM Controller/2(S) -> Gate driver/1(S)
  Sensor rotor/3(w) -> Bus Creator/1  "w"
  connections:
  Inertia/LConn1 -- R/RConn1 -- Sensor rotor/RConn1
  Meas I/RConn1 -- IPMSM/LConn1
  Converter/LConn2 -- Meas I/LConn1
  Sensor rotor/LConn1 -- IPMSM/RConn1
  C/RConn1 -- Converter/RConn2 -- Meas V/RConn1 -- -/RConn1
  Gate driver/RConn1 -- Converter/LConn1
  MRRef/LConn1 -- IPMSM/RConn2
  C/LConn1 -- +/RConn1 -- Converter/RConn1 -- Meas V/LConn1

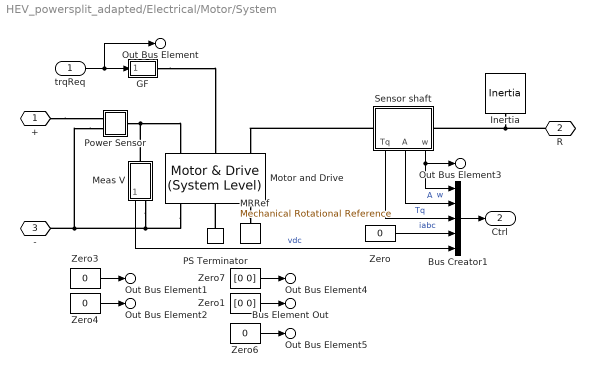
== system HEV_powersplit_adapted/Electrical/Motor/System ==
  trqReq : Inport
  Bus Creator1 : BusCreator  Inputs=5
  GF : Subsystem
      mask Display: disp('GF')
  Inertia : fl_lib/Mechanical/Rotational Elements/Inertia  inertia=HEV_Param.Motor.Shaft_Inertia kg*m^2  num_ports=foundation.enum.numPorts2.one  w_specify=on  w_priority=High  w=0 rad/s  w_nominal_specify=off  w_nominal_value=1  w_nominal_unit=rad/s  t_specify=off  t_priority=High  t=0 N*m  t_nominal_specify=off  t_nominal_value=1  t_nominal_unit=N*m
  MRRef : fl_lib/Mechanical/Rotational Elements/Mechanical Rotational Reference
  Meas V : Subsystem
  Motor and Drive : ee_lib/Electromechanical/Motor & Drive (System Level)  torque_speed_param=1  overtorque_param=ee.enum.electromech.overtorque.no  T_t=HEV_Param.Motor.TorqSpdLUT.TorqueNm N*m  T_t_intermittent=[.36, .32, .28, 0] N*m  T_t_2D=[.09, .09, .09; .08, .08, .08; .07, .07, .07; 0, 0, 0] N*m  T_t_intermittent_2D=[.36, .36, .36; .32, .32, .32; .28, .28, .28; 0, 0, 0] N*m  w_t=HEV_Param.Motor.TorqSpdLUT.SpeedRPM rpm  vdc_t=[6, 12, 24] V  torque_max=0.1 N*m  power_max=30 W  torque_max_intermittent=0.4 N*m  power_max_intermittent=120 W  time_overtorque=30 s  time_recover=60 s  Tc=HEV_Param.Motor.TorqueControl_TimeConst/2 s  EnableSwitch=simscape.enum.onoff.off  losses_param=1  eff=HEV_Param.Motor.Efficiency  w_eff=2000 rpm  T_eff=200 N*m  Piron=0 W  Pbase=0 W  w_eff_vec=[-8000 -4000 0 4000 8000] rpm  T_eff_vec=[0 0.03 0.06 0.09] N*m  v_eff_vec=[100, 250, 400] V  losses_mat=[1.49 1.67 2.21 3.10; 0.42 0.69 1.14 2.03; 0.06 0.24 0.78 1.68; 0.42 0.69 1.14 2.03; 1.49 1.67 2.21 3.10] W  efficiency_mat=[95 95 95 95; 95 95 95 95; 95 95 95 95; 95 95 95 95; 95 95 95 95]  losses_mat_3D=ones(5, 4, 3) W  efficiency_mat_3D=95 * ones(5, 4, 3)  Res=HEV_Param.Motor.Series_Resistance Ohm  J=0 kg*m^2  lam=HEV_Param.Motor.Damping N*m/(rad/s)  speed0=0 rpm  faulted_specify=off  faulted_priority=None  faulted=0  faulted_nominal_specify=off  faulted_nominal_value=1  faulted_nominal_unit=1  isSwitchedOff_specify=off  isSwitchedOff_priority=None  isSwitchedOff=0  isSwitchedOff_nominal_specify=off  isSwitchedOff_nominal_value=1  isSwitchedOff_nominal_unit=1  torqueLimitContinuous_specify=off  torqueLimitContinuous_priority=None  torqueLimitContinuous=0 N*m  torqueLimitContinuous_nominal_specify=off  torqueLimitContinuous_nominal_value=1  torqueLimitContinuous_nominal_unit=N*m  TabulateLossesForMultipleTemperatures=false  alpha=3.93e-3 1/K  Tmeas=25 degC  TmeasVec=[25, 75, 125] degC  Tmeas2=125 degC  losses_mat_T2=[1.49, 1.74, 2.49, 3.74; .42, .67, 1.42, 2.67; .06, .31, 1.06, 2.31; .42, .67, 1.42, 2.67; 1.49, 1.74, 2.49, 3.74] W  efficiency_mat_T2=[95, 95, 95, 95; 95, 95, 95, 95; 95, 95, 95, 95; 95, 95, 95, 95; 95, 95, 95, 95]  losses_mat_3D_T2=ones(5, 4, 3) W  efficiency_mat_3D_T2=95 * ones(5, 4, 3)  lossesMatMultipleTemperatures=ones(5, 4, 3) W  efficiencyMatMultipleTemperatures=95 * ones(5, 4, 3)  lossesMat4DMultipleTemperatures=ones(5, 4, 3, 3) W  efficiencyMat4DMultipleTemperatures=95 * ones(5, 4, 3, 3)  thermal_mass=100 J/K  initial_temperature=25 degC
  PS Terminator : fl_lib/Physical Signals/Sinks/PS Terminator
  Power Sensor : Subsystem
      mask Display: disp('S')
  Sensor shaft : Subsystem
      settings: PortSchema="{\"entries\":[{\"content\":{\"sides\":[{\"content\":{\"connectorIds\":[\"LConn1\"]},\"type\":\"ConnectorPlacement.EquallySpacedRectSide\",\"uuid\":\"0db9bac0-0ae1-4d98-a677-466f391c258c\"},{\"content\":{\"connectorIds\":[\"RConn1\"],\"side\":\"RIGHT\"},\"type\":\"ConnectorPlacement.EquallySpacedRectSide\",\"uuid\":\"8934243c-3b81-4e7c-b06c-d9d72f311b85\"},{\"content\":{\"side\":\"TOP\"},\"type\":\"ConnectorPlacement.EquallySpacedRectSide\",\"uuid\":\"85d02103-2e2c-4b6a-97e8-ffc8c956f28d\"},{\"content\":{\"connectorIds\":[\"Out1\",\"Out2\",\"Out3\"],\"side\":\"BOTTOM\"},\"type\":\"ConnectorPlacement.EquallySpacedRectSide\",\"uuid\":\"2e7d2385-134f-4bd8-b3f4-60582ce11538\"}]},\"type\":\"ConnectorPlacement.EquallySpacedConnector\",\"uuid\":\"45a37dc1-16bf-4b9c-909e-727af625c5bc\"}],\"packageUris\":[\"http://schema.mathworks.com/mf0/Connector/R2020b\"],\"version\":\"1.0\"}"
  Zero{,3..4,6} (4 alike) : Constant  Value=0  OutDataTypeStr=Inherit: Inherit via back propagation
  Zero1 : Constant  Value=[0 0]  OutDataTypeStr=Inherit: Inherit via back propagation
  Zero7 : Constant  Value=[0 0]  OutDataTypeStr=Inherit: Inherit via back propagation
  + : PMIOPort  Side=Left
  R : PMIOPort  Port=2  Side=Right
  - : PMIOPort  Port=3  Side=Left
  Bus Element Out : Outport  PortName=meas  Element=idqRef
  Out Bus Element : Outport  PortName=meas  Element=TqRef
  Out Bus Element1 : Outport  PortName=meas  Element=TqLim
  Out Bus Element2 : Outport  PortName=meas  Element=TqEstim
  Out Bus Element3 : Outport  PortName=meas  Element=Spd
  Out Bus Element5 : Outport  PortName=meas  Element=iabc
  Out Bus Element4 : Outport  PortName=meas  Element=idq
  Ctrl : Outport  Port=2  VectorParamsAs1DForOutWhenUnconnected=off
  wires:
  Zero/1 -> Bus Creator1/4  "iabc"
  Sensor shaft/3(w) -> Out Bus Element3/1, Bus Creator1/1  "w"
  Sensor shaft/1(Tq) -> Bus Creator1/3  "Tq"
  Sensor shaft/2(A) -> Bus Creator1/2  "A"
  Meas V/1(Vdc) -> Bus Creator1/5  "vdc"
  Bus Creator1/1 -> Ctrl/1
  Zero1/1 -> Bus Element Out/1
  trqReq/1 -> Out Bus Element/1, GF/1(In1)
  Zero3/1 -> Out Bus Element1/1
  Zero4/1 -> Out Bus Element2/1
  Zero6/1 -> Out Bus Element5/1
  Zero7/1 -> Out Bus Element4/1
  connections:
  R/RConn1 -- Inertia/LConn1 -- Sensor shaft/RConn1
  PS Terminator/LConn1 -- Motor and Drive/RConn2
  Power Sensor/LConn2 -- Meas V/RConn1 -- Motor and Drive/RConn1 -- -/RConn1
  +/RConn1 -- Power Sensor/LConn1
  Power Sensor/RConn1 -- Meas V/LConn1 -- Motor and Drive/LConn1
  GF/RConn1 -- Motor and Drive/LConn2
  Motor and Drive/RConn3 -- MRRef/LConn1
  Sensor shaft/LConn1 -- Motor and Drive/LConn3

== system HEV_powersplit_adapted/Electrical/Generator/Detailed/Gate driver ==
  S : Inport
  Demux : Demux  Outputs=6
  Simulink-PS Converter{1..6} (6 alike) : nesl_utility/Simulink-PS Converter  PhysicalDomain=network_engine_domain  SubClassName=ps_input  LeftPortType=input  RightPortType=output  PseudoPeriodic=off  Frequencies=[]  NoiseDistribution=none  NoiseParameters=[]  Unit=1  AffineConversion=off  FilteringAndDerivatives=zero  SimscapeFilterOrder=1  InputFilterTimeConstant=0.001  UdotUserProvided=1
  Six-Pulse Gate Multiplexer : ee_lib/Semiconductors & Converters/Converters/Six-Pulse Gate Multiplexer  port_option=ee.enum.controlport.ps
  G : PMIOPort  Side=Right
  wires:
  Demux/1 -> Simulink-PS Converter1/1
  S/1 -> Demux/1
  Demux/4 -> Simulink-PS Converter4/1
  Demux/2 -> Simulink-PS Converter2/1
  Demux/3 -> Simulink-PS Converter3/1
  Demux/5 -> Simulink-PS Converter5/1
  Demux/6 -> Simulink-PS Converter6/1
  connections:
  Six-Pulse Gate Multiplexer/RConn1 -- G/RConn1
  Simulink-PS Converter1/RConn1 -- Six-Pulse Gate Multiplexer/LConn1
  Simulink-PS Converter3/RConn1 -- Six-Pulse Gate Multiplexer/LConn3
  Simulink-PS Converter5/RConn1 -- Six-Pulse Gate Multiplexer/LConn5
  Simulink-PS Converter6/RConn1 -- Six-Pulse Gate Multiplexer/LConn6
  Simulink-PS Converter4/RConn1 -- Six-Pulse Gate Multiplexer/LConn4
  Simulink-PS Converter2/RConn1 -- Six-Pulse Gate Multiplexer/LConn2

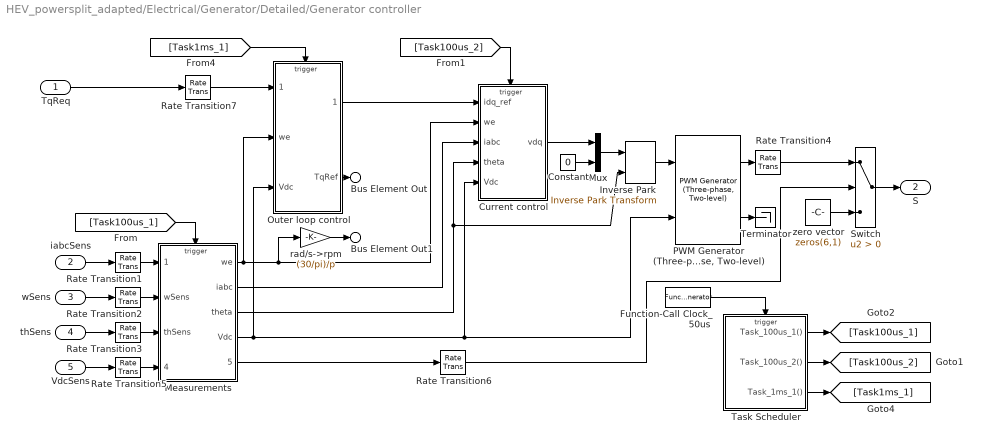
== system HEV_powersplit_adapted/Electrical/Generator/Detailed/Generator controller ==
  TqReq : Inport
  iabcSens : Inport  Port=2
  wSens : Inport  Port=3
  thSens : Inport  Port=4
  VdcSens : Inport  Port=5
  Constant : Constant  Value=0  SampleTime=-1
  Current control : Subsystem
  Function-Call Clock_50us : FunctionCallGenerator  SampleTime=5e-5
  Inverse Park : eeTransforms/Inverse Park Transform  AxisAlignment=Q-axis  PowerInvariant=off
  Measurements : Subsystem
  Mux : Mux  Inputs=2
  Outer loop control : Subsystem
  "PWM Generator (Three-phase, Two-level)" : eePwmGeneratorTwoLevel/PWM Generator (Three-phase, Two-level)  PWMMode=Continuous PWM (CPWM)  CPWMMode=SVM: space vector modulation  DPWMMode=60 DPWM: 60 degree discontinuous PWM  fsw=fsw  Ts=Ts
  Rate Transition{1..7} (7 alike) : RateTransition
  Switch : Switch  Criteria=u2 > Threshold  SaturateOnIntegerOverflow=off  InputSameDT=off
  Task Scheduler : Stateflow chart  TreatAsAtomicUnit=on
  Terminator : Terminator
  rad/s->rpm : Gain  Gain=(30/pi)/p
  zero vector : Constant  Value=zeros(6,1)  SampleTime=-1
  Bus Element Out : Outport  PortName=visGen  Element=TqRef
  Bus Element Out1 : Outport  PortName=visGen  Element=Spd
  S : Outport  Port=2  VectorParamsAs1DForOutWhenUnconnected=off
  wires:
  Rate Transition2/1 -> Measurements/2(wSens)
  VdcSens/1 -> Rate Transition5/1
  wSens/1 -> Rate Transition2/1
  zero vector/1 -> Switch/3
  Measurements/2(iabc) -> Current control/3(iabc)
  [Task100us_1] -> Measurements/Trigger
  Rate Transition1/1 -> Measurements/1(iabcSens)
  Switch/1 -> S/1
  [Task1ms_1] -> Outer loop control/Trigger
  Rate Transition3/1 -> Measurements/3(thSens)
  Outer loop control/1(idqRef) -> Current control/1(idq_ref)
  Measurements/5(PwmEnable) -> Rate Transition6/1
  Task Scheduler/3(Task_1ms_1()) -> [Task1ms_1]
  Measurements/1(we) -> rad/s->rpm/1, Current control/2(we), Outer loop control/2(we)
  Task Scheduler/1(Task_100us_1()) -> [Task100us_1]
  iabcSens/1 -> Rate Transition1/1
  "PWM Generator (Three-phase, Two-level)"/1 -> Rate Transition4/1
  Measurements/3(theta) -> Current control/4(theta), Inverse Park/2
  thSens/1 -> Rate Transition3/1
  Rate Transition6/1 -> Switch/2
  Rate Transition7/1 -> Outer loop control/1(TqReq)
  Task Scheduler/2(Task_100us_2()) -> [Task100us_2]
  Rate Transition5/1 -> Measurements/4(VdcSens)
  "PWM Generator (Three-phase, Two-level)"/2 -> Terminator/1
  Measurements/4(Vdc) -> Outer loop control/3(Vdc), "PWM Generator (Three-phase, Two-level)"/2, Current control/5(Vdc)
  [Task100us_2] -> Current control/Trigger
  Function-Call Clock_50us/1 -> Task Scheduler/Trigger
  Rate Transition4/1 -> Switch/1
  Inverse Park/1 -> "PWM Generator (Three-phase, Two-level)"/1
  Constant/1 -> Mux/2
  Current control/1(vdq) -> Mux/1
  Mux/1 -> Inverse Park/1
  Outer loop control/2(TqRef) -> Bus Element Out/1
  rad/s->rpm/1 -> Bus Element Out1/1
  TqReq/1 -> Rate Transition7/1

== system HEV_powersplit_adapted/Electrical/Generator/Detailed/Meas V ==
  PS-Simulink Converter4 : nesl_utility/PS-Simulink Converter  PhysicalDomain=network_engine_domain  SubClassName=ps_output  LeftPortType=input  RightPortType=output  PseudoPeriodic=off  Frequencies=[]  VectorFormat=1-D array  Unit=V  AffineConversion=off
  Voltage Sensor : fl_lib/Electrical/Electrical Sensors/Voltage Sensor
  - : PMIOPort  Side=Right
  + : PMIOPort  Port=2  Side=Left
  Vdc : Outport  VectorParamsAs1DForOutWhenUnconnected=off
  wires:
  PS-Simulink Converter4/1 -> Vdc/1
  connections:
  PS-Simulink Converter4/LConn1 -- Voltage Sensor/RConn1
  Voltage Sensor/LConn1 -- +/RConn1
  Voltage Sensor/RConn2 -- -/RConn1

== system HEV_powersplit_adapted/Electrical/Generator/Detailed/Sensor iabc ==
  Current Sensor : ee_lib/Sensors & Transducers/Current Sensor (Three-Phase)
  PS-Simulink Converter : nesl_utility/PS-Simulink Converter  PhysicalDomain=network_engine_domain  SubClassName=ps_output  LeftPortType=input  RightPortType=output  PseudoPeriodic=off  Frequencies=[]  VectorFormat=1-D array  Unit=A  AffineConversion=off
  1 : PMIOPort  Side=Left
  2 : PMIOPort  Port=2  Side=Right
  iabc : Outport  VectorParamsAs1DForOutWhenUnconnected=off
  wires:
  PS-Simulink Converter/1 -> iabc/1
  connections:
  1/RConn1 -- Current Sensor/LConn1
  2/RConn1 -- Current Sensor/RConn2
  Current Sensor/RConn1 -- PS-Simulink Converter/LConn1

== system HEV_powersplit_adapted/Electrical/Generator/Detailed/Sensor shaft ==
  MRRef : fl_lib/Mechanical/Rotational Elements/Mechanical Rotational Reference
  Motion Sensor : fl_lib/Mechanical/Mechanical Sensors/Ideal Rotational Motion Sensor  reference=foundation.enum.MeasurementReference.difference  acceleration_port=false  velocity_port=true  position_port=true  wrap_angle=simscape.enum.onoff.off  offset=0 deg
  PS-Simulink Converter1 : nesl_utility/PS-Simulink Converter  PhysicalDomain=network_engine_domain  SubClassName=ps_output  LeftPortType=input  RightPortType=output  PseudoPeriodic=off  Frequencies=[]  VectorFormat=1-D array  Unit=rad/s  AffineConversion=off
  PS-Simulink Converter2 : nesl_utility/PS-Simulink Converter  PhysicalDomain=network_engine_domain  SubClassName=ps_output  LeftPortType=input  RightPortType=output  PseudoPeriodic=off  Frequencies=[]  VectorFormat=1-D array  Unit=rad  AffineConversion=off
  PS-Simulink Converter3 : nesl_utility/PS-Simulink Converter  PhysicalDomain=network_engine_domain  SubClassName=ps_output  LeftPortType=input  RightPortType=output  PseudoPeriodic=off  Frequencies=[]  VectorFormat=1-D array  Unit=N*m  AffineConversion=off
  Torque Sensor : fl_lib/Mechanical/Mechanical Sensors/Ideal Torque Sensor
  R : PMIOPort  Side=Left
  C : PMIOPort  Port=2  Side=Right
  Tq : Outport  VectorParamsAs1DForOutWhenUnconnected=off
  A : Outport  Port=2  VectorParamsAs1DForOutWhenUnconnected=off
  w : Outport  Port=3  VectorParamsAs1DForOutWhenUnconnected=off
  wires:
  PS-Simulink Converter3/1 -> Tq/1
  PS-Simulink Converter1/1 -> w/1
  PS-Simulink Converter2/1 -> A/1
  connections:
  Motion Sensor/RConn2 -- PS-Simulink Converter1/LConn1
  Motion Sensor/RConn1 -- MRRef/LConn1
  R/RConn1 -- Torque Sensor/LConn1
  Torque Sensor/RConn1 -- C/RConn1 -- Motion Sensor/LConn1
  Torque Sensor/RConn2 -- PS-Simulink Converter3/LConn1
  Motion Sensor/RConn3 -- PS-Simulink Converter2/LConn1
